simulink model "OMSv1_3"  (Simulink 6.6)
settings: Solver=ode4  SolverMode=SingleTasking  StartTime=0.0  StopTime=9  FixedStep=0.001  MaxStep=0.001  RelTol=1e-3  AbsTol=1e-3
undefined symbols (not defined in the file): alexlaw, bs_onoff, bs_scale, bsfsacrit, bsfsvcrit, cnsgain, fs_onoff, fs_scale, fsdelaycalc, ltdrk, phasicgain, pmcgain, pmctau2, pmctau3, saccsw, spgain, tonicgain, tvrD, tvrN
(part 2 of 7)

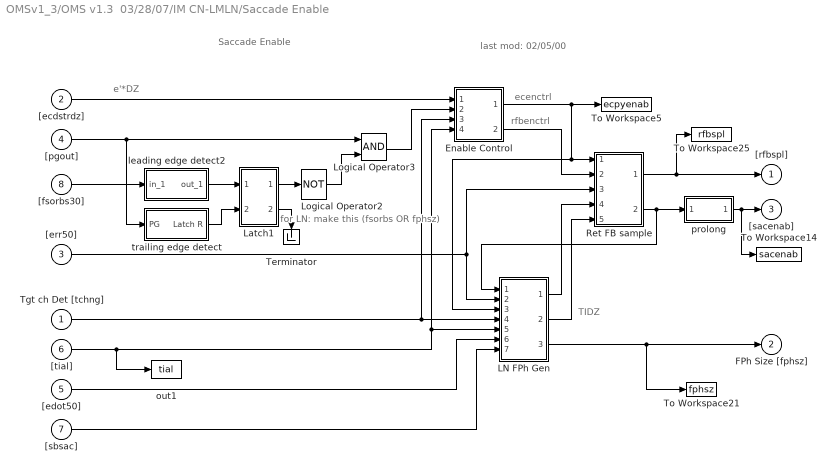
== system OMSv1_3/OMS v1.3  03/28/07/IM CN-LMLN/Saccade Enable ==
  note: Saccade Enable
  note: last mod:
      | 02/05/00
  note: rfbenctrl
  note: ecenctrl
  note: e'*DZ
  note: for LN: make this
      | (fsorbs OR fphsz)
  note: TIDZ
  Tgt ch Det [tchng] : Inport
  "[ecdstrdz]" : Inport  Port=2
  "[err50]" : Inport  Port=3
  "[pgout]" : Inport  Port=4
  "[edot50]" : Inport  Port=5
  "[tial]" : Inport  Port=6
  "[sbsac]" : Inport  Port=7
  "[fsorbs30]" : Inport  Port=8
  Enable Control : Subsystem
      mask Display: disp('Enable\nControl')
  LN FPh Gen : Subsystem
      mask Display: disp('DFFPh\nGen')
  Latch1 : Subsystem  mask(Latch){@1=0}
      mask prompts: @1 "Initial State for Output "Q":"
      mask help: Latch
      mask init:
      | ini=(@1~=0);
      mask Help: Latches the S input.  When S (set) is one, the Q output  becomes one.  The output remains one until the R (reset) input becomes one, forcing the output to zero.  If both R and S are one, the latch will be in an undefined state.
      mask Display: disp('S   Q\n\nR  !Q')
  Logical Operator2 : Logic  Operator=NOT  Inputs=1
  Logical Operator3 : Logic
  Ret FB sample : Subsystem
      mask Display: disp('Ret FB\nEnab &\nSample')
  Terminator : Terminator
      settings: Orientation=down
  To Workspace14 : ToWorkspace  VariableName=sacenab  SaveFormat=Array
      settings: MaxDataPoints=10000
      mask Type: imsw1in
  To Workspace21 : ToWorkspace  VariableName=fphsz  SaveFormat=Array
      settings: MaxDataPoints=10000
  To Workspace25 : ToWorkspace  VariableName=rfbspl  SaveFormat=Array
      settings: MaxDataPoints=10000
      mask Type: imsw1in
  To Workspace5 : ToWorkspace  VariableName=ecpyenab  SaveFormat=Array
      settings: MaxDataPoints=10000
      mask Type: imsw1in
  leading edge detect2 : Subsystem
      mask Display: disp('Leading\nEdge Det')
  out1 : ToWorkspace  VariableName=tial  SaveFormat=Array
      settings: MaxDataPoints=100000
  prolong : Subsystem  mask{prolong=10}
      mask prompts: prolong "Prolong pulse by?  (msec)"
      mask Display: disp('prolong')
  trailing edge detect : Subsystem
      mask Display: disp('Trailing\nEdge Det')
  "[rfbspl]" : Outport  InitialOutput=0
  FPh Size [fphsz] : Outport  Port=2  InitialOutput=0
  "[sacenab]" : Outport  Port=3  InitialOutput=0
  wires:
  "[pgout]"/1 -> Logical Operator3/1, trailing edge detect/1(PG)
  Logical Operator2/1 -> Logical Operator3/2
  "[ecdstrdz]"/1 -> Enable Control/1(e'*DZ [ecdstrdz])
  Tgt ch Det [tchng]/1 -> LN FPh Gen/4(TCD [tchng]), Enable Control/3(Tgt ch Det [tchng])
  "[sbsac]"/1 -> LN FPh Gen/7("[sbsac]")
  "[edot50]"/1 -> LN FPh Gen/6("[edot50]")
  Enable Control/1(ECPY EnTmng [ecpyenab]) -> LN FPh Gen/3("[ecpyenab]"), Ret FB sample/1("[ecpyenab]"), To Workspace5/1
  "[err50]"/1 -> LN FPh Gen/2("[err50]"), Ret FB sample/3("[err50]")
  Enable Control/2(RetFB En&Spl) -> Ret FB sample/2("[rfbenctrl]")
  LN FPh Gen/2(TIDZ) -> Ret FB sample/5(TIDZ)
  Ret FB sample/2(RetFB Enable [sacenab]) -> prolong/1(value(in)), LN FPh Gen/1("[rfbenab]")
  "[fsorbs30]"/1 -> leading edge detect2/1(in_1)
  leading edge detect2/1(out_1) -> Latch1/1(in_1)
  Latch1/1(out_1) -> Logical Operator2/1
  trailing edge detect/1(Latch R) -> Latch1/2(in_2)
  Logical Operator3/1 -> Enable Control/2(VolPG ( [pgout] &NOT fs or bs))
  LN FPh Gen/1("[eedot]") -> Ret FB sample/4("[eedot]")
  Ret FB sample/1(RFB Spl [rfbspl]) -> "[rfbspl]"/1, To Workspace25/1
  LN FPh Gen/3(FPh Size [fphsz]) -> FPh Size [fphsz]/1, To Workspace21/1
  prolong/1(value(out)) -> "[sacenab]"/1, To Workspace14/1
  "[tial]"/1 -> LN FPh Gen/5("[tial]"), Enable Control/4("[tial]"), out1/1
  Latch1/2(out_2) -> Terminator/1

== system OMSv1_3/OMS v1.3  03/28/07/IM CN-LMLN/Saccade Motor Commmand ==
  note: last mod:
      | 02/25/01
  note: Saccadic Motor Command
  note: If TCHNG occurs, BLOCK
      | BS/FS (and already prog vs?)
      | for 150 msec
  note: If TCHNG occurs:
      | ALLOW vol sacc
  note: make sure that tchngOVR
      | lets _something_ pass,
      | since it operates switches
      | in two different locations...
  "[ecdstrdz]" : Inport
  "[fphsz]" : Inport  Port=2
  Tgt ch Det [tchng] : Inport  Port=3
  "[sacenab]" : Inport  Port=4
  "[fsorbs30]" : Inport  Port=5
  "[fsbcmc30]" : Inport  Port=6
  "\"slip vel\"1" : Sum  SaturateOnIntegerOverflow=on  InputSameDT=on
  (0.5) : Switch  Threshold=.5  SaturateOnIntegerOverflow=on  InputSameDT=on
  0 : Constant  Orientation=left  Value=0
  Switch3 : Switch  Threshold=.5  SaturateOnIntegerOverflow=on  InputSameDT=on
  TCHNG Override : Subsystem
      mask Display: disp('TCHNG\nOverride')
  To Workspace30 : ToWorkspace  VariableName=fsbsmc30  SaveFormat=Array
      settings: MaxDataPoints=10000
  To Workspace6 : ToWorkspace  VariableName=posmc  SaveFormat=Array
      settings: MaxDataPoints=10000
  Voluntary Saccade Switch : Subsystem
      mask Display: disp('Vol\nSacc\nSw')
  timer value : Constant  Orientation=left  Value=0.15
  "[posmc]" : Outport  InitialOutput=0
  wires:
  "[ecdstrdz]"/1 -> "\"slip vel\"1"/1
  "[fphsz]"/1 -> "\"slip vel\"1"/2
  "[sacenab]"/1 -> Voluntary Saccade Switch/2("[sacenab]")
  0/1 -> Switch3/3
  (0.5)/1 -> Switch3/1
  "[fsorbs30]"/1 -> Voluntary Saccade Switch/3("[fsorbs30]")
  Voluntary Saccade Switch/2(sacenab/0) -> (0.5)/2
  Tgt ch Det [tchng]/1 -> TCHNG Override/1("[tchng]")
  timer value/1 -> TCHNG Override/2(timer dur)
  "\"slip vel\"1"/1 -> Voluntary Saccade Switch/1("[fphmag]")
  Voluntary Saccade Switch/1("[vsmc]") -> (0.5)/1
  TCHNG Override/1(tchng sw) -> Switch3/2
  "[fsbcmc30]"/1 -> (0.5)/3, To Workspace30/1
  Switch3/1 -> "[posmc]"/1, To Workspace6/1

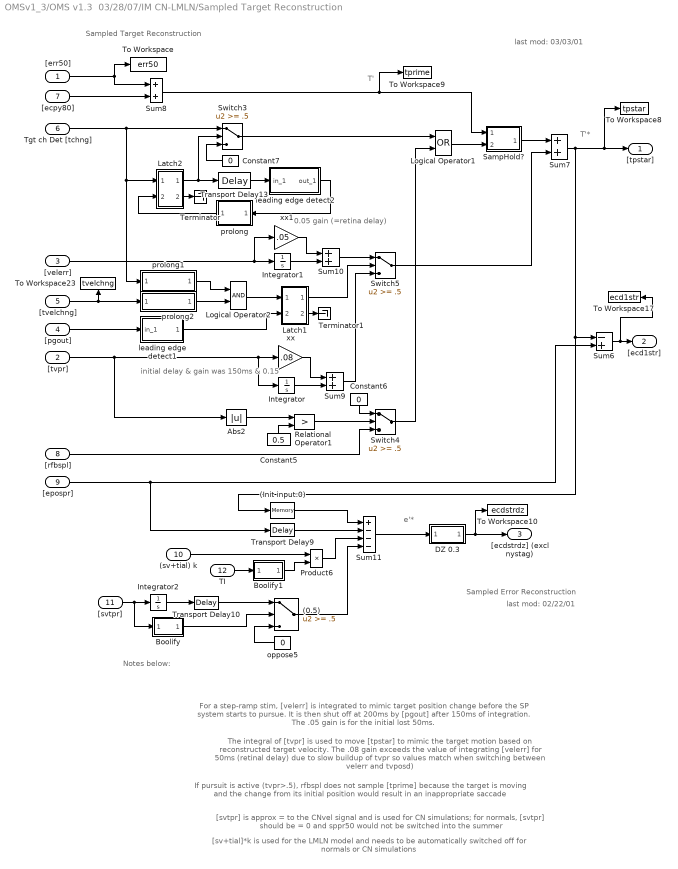
== system OMSv1_3/OMS v1.3  03/28/07/IM CN-LMLN/Sampled Target Reconstruction ==
  note: T'
  note: T'*
  note: Sampled Target Reconstruction
  note: last mod:
      | 03/03/01
  note: Notes below:
  note: If pursuit is active (tvpr>.5), rfbspl does not sample [tprime] because the target is moving and
      | the change from its initial position would result in an inappropriate saccade
  note: The integral of [tvpr] is used to move [tpstar] to mimic the target motion based on reconstructed target velocity. The .08 gain
      | exceeds the value of integrating [velerr] for 50ms (retinal delay) due to slow buildup of tvpr so values match
      | when switching between velerr and tvposd)
  note: For a step-ramp stim, [velerr] is integrated to mimic target position change before the SP system starts to pursue.
      |  It is then shut off at 200ms by [pgout] after 150ms of integration. The .05 gain is for the initial lost 50ms.
  note: initial delay & gain
      | was 150ms & 0.15
  note: 0.05 gain (=retina delay)
  note: e'*
  note: Sampled Error Reconstruction
  note: last mod:
      | 02/22/01
  note: [svtpr] is approx = to the CNvel signal and is used for CN simulations; for normals, [svtpr]
      | should be = 0 and sppr50 would not be switched into the summer
  note: [sv+tial]*k is used for the LMLN model and needs to be automatically switched off
      | for normals or CN simulations
  "[err50]" : Inport
  "[tvpr]" : Inport  Port=2
  "[velerr]" : Inport  Port=3
  "[pgout]" : Inport  Port=4
  "[tvelchng]" : Inport  Port=5
  Tgt ch Det [tchng] : Inport  Port=6
  "[ecpy80]" : Inport  Port=7
  "[rfbspl]" : Inport  Port=8
  "[epospr]" : Inport  Port=9
  (sv+tial) k : Inport  Port=10
  "[svtpr]" : Inport  Port=11
  TI : Inport  Port=12
  (0.5) : Switch  Threshold=.5  SaturateOnIntegerOverflow=on  InputSameDT=on
  (Init input:0) : Memory
  Abs2 : Abs  SaturateOnIntegerOverflow=on
  Boolify : Subsystem
      mask Display: disp('Boolify')
  Boolify1 : Subsystem
      mask Display: disp('Boolify')
  Constant5 : Constant  Orientation=up  Value=0.5
  Constant6 : Constant  Orientation=down  Value=0
  Constant7 : Constant  Orientation=left  Value=0
  DZ 0.3 : Subsystem
      mask Display: disp('DZ 0.3')
  Integrator : Integrator
  Integrator1 : Integrator
  Integrator2 : Integrator
  Latch1 : Subsystem  mask(Latch){@1=0}
      mask prompts: @1 "Initial State for Output "Q":"
      mask help: Latch
      mask init:
      | ini=(@1~=0);
      mask Help: Latches the S input.  When S (set) is one, the Q output  becomes one.  The output remains one until the R (reset) input becomes one, forcing the output to zero.  If both R and S are one, the latch will be in an undefined state.
      mask Display: disp('S   Q\n\nR  !Q')
  Latch2 : Subsystem  mask(Latch){@1=0}
      mask prompts: @1 "Initial State for Output "Q":"
      mask help: Latch
      mask init:
      | ini=(@1~=0);
      mask Help: Latches the S input.  When S (set) is one, the Q output  becomes one.  The output remains one until the R (reset) input becomes one, forcing the output to zero.  If both R and S are one, the latch will be in an undefined state.
      mask Display: disp('S   Q\n\nR  !Q')
  Logical Operator1 : Logic  Operator=OR
  Logical Operator2 : Logic
  Product6 : Product  SaturateOnIntegerOverflow=on  RndMeth=Zero  InputSameDT=on
  Relational Operator1 : RelationalOperator  Operator=>  InputSameDT=on
  SampHold? : Subsystem
      mask Display: disp('S=H\nH=L')
  Sum{7..10} (4 alike) : Sum  SaturateOnIntegerOverflow=on  InputSameDT=on
  Sum11 : Sum  Inputs=+---  SaturateOnIntegerOverflow=on  InputSameDT=on
  Sum6 : Sum  Inputs=-+  SaturateOnIntegerOverflow=on  InputSameDT=on
  Switch3 : Switch  Threshold=.5  SaturateOnIntegerOverflow=on  InputSameDT=on
  Switch4 : Switch  Threshold=.5  SaturateOnIntegerOverflow=on  InputSameDT=on
  Switch5 : Switch  Threshold=.5  SaturateOnIntegerOverflow=on  InputSameDT=on
  Terminator : Terminator
  Terminator1 : Terminator
  To Workspace : ToWorkspace  VariableName=err50  SaveFormat=Array
      settings: MaxDataPoints=10000
  To Workspace10 : ToWorkspace  VariableName=ecdstrdz  SaveFormat=Array
      settings: MaxDataPoints=10000
  To Workspace17 : ToWorkspace  VariableName=ecd1str  SaveFormat=Array
      settings: MaxDataPoints=10000
  To Workspace23 : ToWorkspace  VariableName=tvelchng  SaveFormat=Array
      settings: Orientation=up  MaxDataPoints=10000
  To Workspace8 : ToWorkspace  VariableName=tpstar  SaveFormat=Array
      settings: MaxDataPoints=10000
  To Workspace9 : ToWorkspace  VariableName=tprime  SaveFormat=Array
      settings: MaxDataPoints=10000
  Transport Delay10 : TransportDelay  DelayTime=.05
      mask Display: disp('50ms')
  Transport Delay13 : TransportDelay  DelayTime=.05
      mask Display: disp('50ms')
  Transport Delay9 : TransportDelay  DelayTime=.05
      mask Display: disp('50ms')
  leading edge detect1 : Subsystem
      mask Display: disp('Leading\nEdge Det')
  leading edge detect2 : Subsystem
      mask Display: disp('Leading\nEdge Det')
  oppose5 : Constant  Orientation=left  Value=0
  prolong : Subsystem  Orientation=left  mask{prolong=150}
      mask prompts: prolong "Prolong pulse by?  (msec)"
      mask Display: disp('150ms\nprolong')
  prolong1 : Subsystem  mask{prolong=5}
      mask prompts: prolong "Prolong pulse by?  (msec)"
      mask Display: disp('5ms prolong')
  prolong2 : Subsystem  mask{prolong=5}
      mask prompts: prolong "Prolong pulse by?  (msec)"
      mask Display: disp('5ms prolong')
  xx : Gain  Gain=.08  SaturateOnIntegerOverflow=on
  xx1 : Gain  Gain=.05  SaturateOnIntegerOverflow=on
  "[tpstar]" : Outport  InitialOutput=0
  "[ecd1str]" : Outport  Port=2  InitialOutput=0
  "[ecdstrdz] (excl nystag)" : Outport  Port=3  InitialOutput=0
  wires:
  Sum8/1 -> To Workspace9/1, SampHold?/1(Input)
  "[ecpy80]"/1 -> Sum8/2
  prolong1/1(value(out)) -> Logical Operator2/1
  Tgt ch Det [tchng]/1 -> Switch3/1, Latch2/1(in_1), prolong1/1(value(in))
  Logical Operator1/1 -> SampHold?/2(S/H?)
  Sum7/1 -> Sum6/1, (Init input:0)/1, "[tpstar]"/1, To Workspace8/1
  SampHold?/1(output) -> Sum7/1
  Switch3/1 -> Logical Operator1/1
  Constant7/1 -> Switch3/3
  Latch2/1(out_1) -> Switch3/2, Transport Delay13/1
  Transport Delay13/1 -> leading edge detect2/1(in_1)
  leading edge detect2/1(out_1) -> prolong/1(value(in))
  prolong/1(value(out)) -> Latch2/2(in_2)
  Sum10/1 -> Switch5/1
  Integrator1/1 -> Sum10/2
  xx1/1 -> Sum10/1
  Abs2/1 -> Relational Operator1/1
  Constant6/1 -> Switch4/1
  Constant5/1 -> Relational Operator1/2
  Relational Operator1/1 -> Switch4/2
  "[rfbspl]"/1 -> Switch4/3
  Integrator/1 -> Sum9/2
  xx/1 -> Sum9/1
  "[tvpr]"/1 -> Abs2/1, xx/1, Integrator/1
  Switch4/1 -> Logical Operator1/2
  leading edge detect1/1(out_1) -> Latch1/2(in_2)
  "[pgout]"/1 -> leading edge detect1/1(in_1)
  Logical Operator2/1 -> Latch1/1(in_1)
  prolong2/1(value(out)) -> Logical Operator2/2
  "[velerr]"/1 -> Integrator1/1, xx1/1
  Switch5/1 -> Sum7/2
  Latch1/1(out_1) -> Switch5/2
  Sum9/1 -> Switch5/3
  "[epospr]"/1 -> Sum6/2, Transport Delay9/1
  "[tvelchng]"/1 -> prolong2/1(value(in)), To Workspace23/1
  Sum6/1 -> "[ecd1str]"/1, To Workspace17/1
  "[err50]"/1 -> Sum8/1, To Workspace/1
  TI/1 -> Boolify1/1(In1)
  Boolify1/1(Out1) -> Product6/2
  (sv+tial) k/1 -> Product6/1
  Product6/1 -> Sum11/3
  oppose5/1 -> (0.5)/3
  "[svtpr]"/1 -> Integrator2/1, Boolify/1(In1)
  Boolify/1(Out1) -> (0.5)/2
  (Init input:0)/1 -> Sum11/1
  Transport Delay9/1 -> Sum11/2
  Sum11/1 -> DZ 0.3/1(in_1)
  Transport Delay10/1 -> (0.5)/1
  (0.5)/1 -> Sum11/4
  Integrator2/1 -> Transport Delay10/1
  DZ 0.3/1(out_1) -> "[ecdstrdz] (excl nystag)"/1, To Workspace10/1
  Latch2/2(out_2) -> Terminator/1
  Latch1/2(out_2) -> Terminator1/1

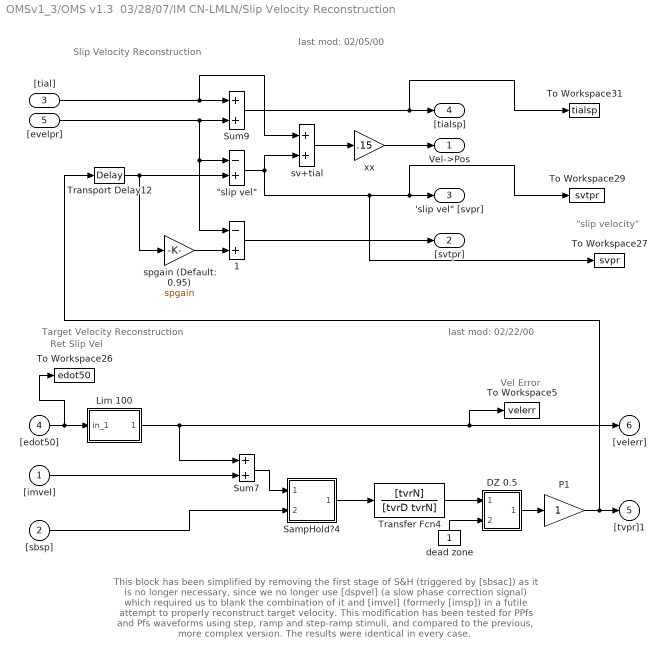
== system OMSv1_3/OMS v1.3  03/28/07/IM CN-LMLN/Slip Velocity Reconstruction ==
  note: last mod:
      | 02/05/00
  note: Slip Velocity Reconstruction
  note: last mod:
      | 02/22/00
  note: Target Velocity Reconstruction
  note: This block has been simplified by removing the first stage of S&H (triggered by [sbsac]) as it is no longer necessary,
      | since we no longer use [dspvel] (a slow phase correction signal) which required us to blank the combination of it
      | and [imvel] (formerly [imsp]) in a futile attempt to properly reconstruct target velocity.  This modification has been tested
      | for PPfs and Pfs waveforms using step, ramp and step-ramp stimuli, and compared to the previous, more complex
      | version.  The results were identical in every case.
  note: "slip velocity"
  note: Vel
      | Error
  note: Ret Slip Vel
  "[imvel]" : Inport
  "[sbsp]" : Inport  Port=2
  "[tial]" : Inport  Port=3
  "[edot50]" : Inport  Port=4
  "[evelpr]" : Inport  Port=5
  " 1" : Sum  Inputs=-+  SaturateOnIntegerOverflow=on  InputSameDT=on
  "\"slip vel\"" : Sum  Inputs=-+  SaturateOnIntegerOverflow=on  InputSameDT=on
  DZ 0.5 : Subsystem
      mask Display: disp('Dead\nZone')
  Lim 100 : Subsystem
      mask Display: disp('Limiter')
  P1 : Gain  SaturateOnIntegerOverflow=on
  SampHold?4 : Subsystem
      mask Display: disp('S=H\nH=L')
  Sum7 : Sum  SaturateOnIntegerOverflow=on  InputSameDT=on
  Sum9 : Sum  SaturateOnIntegerOverflow=on  InputSameDT=on
  To Workspace26 : ToWorkspace  VariableName=edot50  SaveFormat=Array
      settings: MaxDataPoints=10000
  To Workspace27 : ToWorkspace  VariableName=svpr  SaveFormat=Array
      settings: MaxDataPoints=10000
  To Workspace29 : ToWorkspace  VariableName=svtpr  SaveFormat=Array
      settings: MaxDataPoints=10000
  To Workspace31 : ToWorkspace  VariableName=tialsp  SaveFormat=Array
      settings: MaxDataPoints=10000
  To Workspace5 : ToWorkspace  VariableName=velerr  SaveFormat=Array
      settings: MaxDataPoints=10000
  Transfer Fcn4 : TransferFcn  Numerator=[tvrN]  Denominator=[tvrD tvrN]
  Transport Delay12 : TransportDelay  DelayTime=.05
      mask Display: disp('50ms')
  dead zone : Constant  Orientation=up
  spgain (Default: 0.95) : Gain  Gain=spgain  SaturateOnIntegerOverflow=on
  sv+tial : Sum  SaturateOnIntegerOverflow=on  InputSameDT=on
  xx : Gain  Gain=.15  SaturateOnIntegerOverflow=on
  Vel->Pos : Outport  InitialOutput=0
  "[svtpr]" : Outport  Port=2  InitialOutput=0
  "'slip vel\" [svpr]" : Outport  Port=3  InitialOutput=0
  "[tialsp]" : Outport  Port=4  InitialOutput=0
  "[tvpr]1" : Outport  Port=5  InitialOutput=0
  "[velerr]" : Outport  Port=6  InitialOutput=0
  wires:
  xx/1 -> Vel->Pos/1
  sv+tial/1 -> xx/1
  "[tial]"/1 -> sv+tial/1, Sum9/1
  "\"slip vel\""/1 -> sv+tial/2, To Workspace27/1, "'slip vel\" [svpr]"/1, To Workspace29/1
  "[evelpr]"/1 -> Sum9/2, "\"slip vel\""/1, " 1"/1
  spgain (Default: 0.95)/1 -> " 1"/2
  " 1"/1 -> "[svtpr]"/1
  Transport Delay12/1 -> "\"slip vel\""/2, spgain (Default: 0.95)/1
  dead zone/1 -> DZ 0.5/2(in_2)
  DZ 0.5/1(out_1) -> P1/1
  "[sbsp]"/1 -> SampHold?4/2(S/H?)
  "[imvel]"/1 -> Sum7/2
  Lim 100/1(out_1) -> Sum7/1, "[velerr]"/1, To Workspace5/1
  Sum7/1 -> SampHold?4/1(Input)
  SampHold?4/1(output) -> Transfer Fcn4/1
  Transfer Fcn4/1 -> DZ 0.5/1(in_1)
  Sum9/1 -> "[tialsp]"/1, To Workspace31/1
  "[edot50]"/1 -> Lim 100/1(in_1), To Workspace26/1
  P1/1 -> "[tvpr]1"/1, Transport Delay12/1

== system OMSv1_3/OMS v1.3  03/28/07/IM CN-LMLN/Target Change Detection ==
  note: Target Change Detection
  note: Detects T change >1 deg any time
  RetErr Vel [edot50] : Inport
  "[tvpr]" : Inport  Port=2
  Abs2 : Abs  SaturateOnIntegerOverflow=on
  Abs3 : Abs  SaturateOnIntegerOverflow=on
  Constant5 : Constant  Orientation=up  Value=950
  Constant6 : Constant  Orientation=up  Value=950
  Derivative : Derivative
      mask Display: disp('s')
  Relational Operator : RelationalOperator  InputSameDT=on
  Relational Operator1 : RelationalOperator  InputSameDT=on
  To Workspace20 : ToWorkspace  VariableName=tchng  SaveFormat=Array
      settings: MaxDataPoints=10000
  Tvel Chng [tvelchng] : Outport  InitialOutput=0
  Trgt Chng [tchng] : Outport  Port=2  InitialOutput=0
  wires:
  RetErr Vel [edot50]/1 -> Abs2/1
  Constant5/1 -> Relational Operator/2
  Abs2/1 -> Relational Operator/1
  Constant6/1 -> Relational Operator1/2
  Abs3/1 -> Relational Operator1/1
  "[tvpr]"/1 -> Derivative/1
  Derivative/1 -> Abs3/1
  Relational Operator1/1 -> Tvel Chng [tvelchng]/1
  Relational Operator/1 -> Trgt Chng [tchng]/1, To Workspace20/1

== system OMSv1_3/OMS v1.3  03/28/07/IM CN-LMLN/setmdlp ==

== system OMSv1_3/OMS v1.3  03/28/07/OMN2/SampHold? ==
  note: When "S/H?" is LOW, then "Input" is switched directly to the
      | output ("sample").  When "S/H?" is HIGH, the current output is
      | maintained ("hold").
  Input : Inport
  S/H? : Inport  Port=2
  Memory : Memory  Orientation=left
  Sign : Subsystem
      mask Type: Sign
      mask Description: y = sign(x)
      mask Help: Sign Function:\n\t\t\ty = 1 if x > 0\n\t\t\ty = 0 if x = 0\n\t\t\ty = -1 if x < 0
      mask Display: plot(-50,-50,50,50,[-50,50],[0,0],[0,0],[-50,50],[-40,0],[-30,-30],[0,40],[30,30])
  Switch2 : Switch  Threshold=0.5  SaturateOnIntegerOverflow=on  InputSameDT=on
  output : Outport  InitialOutput=0
  wires:
  Switch2/1 -> Memory/1, output/1
  Memory/1 -> Switch2/1
  Input/1 -> Switch2/3
  Sign/1(out_1) -> Switch2/2
  S/H?/1 -> Sign/1(in_1)

== system OMSv1_3/OMS v1.3  03/28/07/OMN2/Sign ==
  in_1 : Inport
  Constant : Constant  Value=0
  Relational Operator : RelationalOperator  Operator=>  InputSameDT=on
  Relational Operator1 : RelationalOperator  Operator=<  InputSameDT=on
  Sum : Sum  Inputs=+-  SaturateOnIntegerOverflow=on  InputSameDT=on
  out_1 : Outport  InitialOutput=0
  wires:
  Sum/1 -> out_1/1
  Relational Operator/1 -> Sum/1
  Relational Operator1/1 -> Sum/2
  Constant/1 -> Relational Operator1/2, Relational Operator/2
  in_1/1 -> Relational Operator/1, Relational Operator1/1

== system OMSv1_3/OMS v1.3  03/28/07/OMS model lib/plantlib link ==

== system OMSv1_3/OMS v1.3  03/28/07/OMS model lib/plantlib link1 ==

== system OMSv1_3/OMS v1.3  03/28/07/OMS model lib/plantlib link2 ==

== system OMSv1_3/OMS v1.3  03/28/07/OMS model lib/plantlib link3 ==

== system OMSv1_3/OMS v1.3  03/28/07/OMS model lib/plantlib link4 ==

== system OMSv1_3/OMS v1.3  03/28/07/OMS model lib/plantlib link5 ==

== system OMSv1_3/OMS v1.3  03/28/07/OMS model lib/plantlib link6 ==

== system OMSv1_3/OMS v1.3  03/28/07/OMS model lib/plantlib link7 ==

== system OMSv1_3/OMS v1.3  03/28/07/OMS model lib/stimlib ==

== system OMSv1_3/OMS v1.3  03/28/07/PG w rNI1/PW funct ==
  note: This process continues until the error has been driven to zero or the input drops to zero,
      | and the integrator is reset and the pulse is ended.
  note: The input, scaled by the piece-wise linear function, is compared to the output of the
      | resettable integrator, which integrates a constant value each iteration.
  note: This block uses a resettable integrator and a piecewise-linear function (PWfunc) to generate
      | a pulse of appropriate duration for the incoming stimulus.
  note: (Init input:0)
  note: PW Function
  mcspl : Inport
  Abs : Abs  SaturateOnIntegerOverflow=on
  Constant1 : Constant  Orientation=up  Value=0
  Constant3 : Constant  Orientation=down  Value=1000
  Good Reset Integrator2 : Subsystem  Orientation=left
      mask Display: disp('Resettable\nNI')
  Input Switch : Subsystem
      mask Display: disp('Input\nSwitch')
  Logical Operator : Logic  Orientation=left  Operator=OR
  Logical Operator1 : Logic  Orientation=up  Operator=NOT  Inputs=1
  PWfn : Lookup  Orientation=down  InputValues=[ 0, 0.1:5, 5:10, 10:50 ]  OutputValues="[ 0, (0.1:5)*0+15,  (5:10)*1+10,  (10:50)*2]"  SaturateOnIntegerOverflow=on
  Relational Operator1 : RelationalOperator  InputSameDT=on
  Relational Operator2 : RelationalOperator  Operator=<=  InputSameDT=on
  Sign : Subsystem
      mask Type: Sign
      mask Description: y = sign(x)
      mask Help: Sign Function:\n\t\t\ty = 1 if x > 0\n\t\t\ty = 0 if x = 0\n\t\t\ty = -1 if x < 0
      mask Display: plot(-50,-50,50,50,[-50,50],[0,0],[0,0],[-50,50],[-40,0],[-30,-30],[0,40],[30,30])
  Sum : Sum  Inputs=-+  SaturateOnIntegerOverflow=on  InputSameDT=on
  dead zone : Constant  Orientation=up  Value=.04
  loop breaker : Memory  Orientation=left
  out thresh : Constant  Value=0.2
  pgw : Outport  InitialOutput=0
  wires:
  Logical Operator1/1 -> Logical Operator/2
  Relational Operator1/1 -> Logical Operator1/1, Sign/1(in_1)
  Constant3/1 -> Good Reset Integrator2/1(input)
  Constant1/1 -> Good Reset Integrator2/3(initial condition)
  out thresh/1 -> Relational Operator1/2
  Input Switch/1(mcsw) -> Abs/1
  mcspl/1 -> Input Switch/1(mcspl)
  Sign/1(out_1) -> pgw/1, loop breaker/1
  Abs/1 -> PWfn/1, Relational Operator2/1
  PWfn/1 -> Sum/2
  Sum/1 -> Relational Operator1/1
  Logical Operator/1 -> Good Reset Integrator2/2(reset?)
  Good Reset Integrator2/1(out_1) -> Sum/1
  dead zone/1 -> Relational Operator2/2
  Relational Operator2/1 -> Logical Operator/1
  loop breaker/1 -> Input Switch/2(pgw)

== system OMSv1_3/OMS v1.3  03/28/07/PG w rNI1/RefLatch (Default = 50ms) ==
  note: It's a cheap trick, but it seems to work:
  note: The falling edge" block's output becomes DISABLED upon
      | detection of the END of the input pulse, and remains
      | so until the refractory period of rp milliseconds has elapsed.
  note: By ANDing these outputs, we get a signal that is DISABLED
      | starting with the beginning of the input pulse, and remains so until
      | rp milliseconds after the termination of the pulse.
  note: The "NOT" gate outputs a DISABLE signal whenever there is any
      | input, so that there can be no response.
  in_1 : Inport
  Abs : Abs  SaturateOnIntegerOverflow=on
  Logical Operator : Logic
  Logical Operator1 : Logic  Operator=NOT  Inputs=1
  trailing edge : Subsystem
      mask Display: disp('Refract\nLatch (te)')
  out_1 : Outport  InitialOutput=0
  wires:
  Logical Operator/1 -> out_1/1
  Logical Operator1/1 -> Logical Operator/1
  trailing edge/1(out_1) -> Logical Operator/2
  Abs/1 -> Logical Operator1/1, trailing edge/1(in_1)
  in_1/1 -> Abs/1

== system OMSv1_3/OMS v1.3  03/28/07/PG w rNI1/SampHold?1 ==
  note: When "S/H?" is HIGH, then "Input" is switched directly to the
      | output ("sample").  When "S/H?" is LOW, the current output is
      | maintained ("hold").
  Input : Inport
  S/H? : Inport  Port=2
  Memory : Memory  Orientation=left
  Sign : Subsystem
      mask Type: Sign
      mask Description: y = sign(x)
      mask Help: Sign Function:\n\t\t\ty = 1 if x > 0\n\t\t\ty = 0 if x = 0\n\t\t\ty = -1 if x < 0
      mask Display: plot(-50,-50,50,50,[-50,50],[0,0],[0,0],[-50,50],[-40,0],[-30,-30],[0,40],[30,30])
  Switch2 : Switch  Threshold=0.5  SaturateOnIntegerOverflow=on  InputSameDT=on
  output : Outport  InitialOutput=0
  wires:
  S/H?/1 -> Sign/1(in_1)
  Sign/1(out_1) -> Switch2/2
  Input/1 -> Switch2/1
  Switch2/1 -> output/1, Memory/1
  Memory/1 -> Switch2/3

== system OMSv1_3/OMS v1.3  03/28/07/Fixation/30 /Latch1 ==
  in_1 : Inport
  in_2 : Inport  Port=2
  Demux : Demux  Outputs=2
  Logic : CombinatorialLogic  TruthTable=[0 1;0 1;1 0;0 1;1 0;0 1;1 0;1 0]
  Memory : Memory  Orientation=left  X0=ini
  Mux : Mux  Inputs=3
  out_1 : Outport  InitialOutput=0
  out_2 : Outport  Port=2  InitialOutput=0
  wires:
  in_2/1 -> Mux/3
  in_1/1 -> Mux/2
  Memory/1 -> Mux/1
  Demux/1 -> Memory/1, out_1/1
  Mux/1 -> Logic/1
  Logic/1 -> Demux/1
  Demux/2 -> out_2/1

== system OMSv1_3/OMS v1.3  03/28/07/Fixation/30 /SampHold?2 ==
  note: When "S/H?" is LOW, then "Input" is switched directly to the
      | output ("sample").  When "S/H?" is HIGH, the current output is
      | maintained ("hold").
  Input : Inport
  S/H? : Inport  Port=2
  Memory : Memory  Orientation=left
  Sign : Subsystem
      mask Type: Sign
      mask Description: y = sign(x)
      mask Help: Sign Function:\n\t\t\ty = 1 if x > 0\n\t\t\ty = 0 if x = 0\n\t\t\ty = -1 if x < 0
      mask Display: plot(-50,-50,50,50,[-50,50],[0,0],[0,0],[-50,50],[-40,0],[-30,-30],[0,40],[30,30])
  Switch2 : Switch  Threshold=0.5  SaturateOnIntegerOverflow=on  InputSameDT=on
  output : Outport  InitialOutput=0
  wires:
  S/H?/1 -> Sign/1(in_1)
  Sign/1(out_1) -> Switch2/2
  Input/1 -> Switch2/3
  Switch2/1 -> Memory/1, output/1
  Memory/1 -> Switch2/1

== system OMSv1_3/OMS v1.3  03/28/07/Fixation/30 /leading edge detect ==
  note: leading edge detection
  in_1 : Inport
  Abs : Abs  SaturateOnIntegerOverflow=on
  Derivative : Derivative
  Relational Operator : RelationalOperator  Operator===  InputSameDT=on
  Sign : Subsystem
      mask Type: Sign
      mask Description: y = sign(x)
      mask Help: Sign Function:\n\t\t\ty = 1 if x > 0\n\t\t\ty = 0 if x = 0\n\t\t\ty = -1 if x < 0
      mask Display: plot(-50,-50,50,50,[-50,50],[0,0],[0,0],[-50,50],[-40,0],[-30,-30],[0,40],[30,30])
  Threshold 1 : Constant
  out_1 : Outport  InitialOutput=0
  wires:
  in_1/1 -> Abs/1
  Relational Operator/1 -> out_1/1
  Threshold 1/1 -> Relational Operator/2
  Sign/1(out_1) -> Relational Operator/1
  Derivative/1 -> Sign/1(in_1)
  Abs/1 -> Derivative/1

== system OMSv1_3/OMS v1.3  03/28/07/Fixation/30 /trailing edge detect ==
  note: It is also possible to remove the SIGNUM function
      | and the '==', and replace them with a simple
      | switch with a threshold of (say) 150 or so.
  note: trailing edge detection
  in_1 : Inport
  Abs : Abs  SaturateOnIntegerOverflow=on
  Derivative : Derivative
  Relational Operator : RelationalOperator  Operator===  InputSameDT=on
  Sign : Subsystem
      mask Type: Sign
      mask Description: y = sign(x)
      mask Help: Sign Function:\n\t\t\ty = 1 if x > 0\n\t\t\ty = 0 if x = 0\n\t\t\ty = -1 if x < 0
      mask Display: plot(-50,-50,50,50,[-50,50],[0,0],[0,0],[-50,50],[-40,0],[-30,-30],[0,40],[30,30])
  Threshold 1 : Constant  Value=-1
  out_1 : Outport  InitialOutput=0
  wires:
  Abs/1 -> Derivative/1
  Derivative/1 -> Sign/1(in_1)
  Sign/1(out_1) -> Relational Operator/1
  Threshold 1/1 -> Relational Operator/2
  Relational Operator/1 -> out_1/1
  in_1/1 -> Abs/1

== system OMSv1_3/OMS v1.3  03/28/07/Fixation/Boolify2/direction1 ==
  in_1 : Inport
  Constant : Constant  Value=0
  Relational Operator : RelationalOperator  Operator=>  InputSameDT=on
  Relational Operator1 : RelationalOperator  Operator=<  InputSameDT=on
  Sum : Sum  Inputs=+-  SaturateOnIntegerOverflow=on  InputSameDT=on
  out_1 : Outport  InitialOutput=0
  wires:
  in_1/1 -> Relational Operator/1, Relational Operator1/1
  Constant/1 -> Relational Operator1/2, Relational Operator/2
  Relational Operator1/1 -> Sum/2
  Relational Operator/1 -> Sum/1
  Sum/1 -> out_1/1

== system OMSv1_3/OMS v1.3  03/28/07/IM CN-LMLN/Alexander's Law/Boolify ==
  TI : Inport
  Abs2 : Abs  SaturateOnIntegerOverflow=on
  direction1 : Subsystem
      mask Type: Sign
      mask Description: y = sign(x)
      mask Help: Sign Function:\n\t\t\ty = 1 if x > 0\n\t\t\ty = 0 if x = 0\n\t\t\ty = -1 if x < 0
      mask Display: plot(-50,-50,50,50,[-50,50],[0,0],[0,0],[-50,50],[-40,0],[-30,-30],[0,40],[30,30])
  Switch Control : Outport  InitialOutput=0
  wires:
  direction1/1(out_1) -> Switch Control/1
  TI/1 -> Abs2/1
  Abs2/1 -> direction1/1(in_1)

== system OMSv1_3/OMS v1.3  03/28/07/IM CN-LMLN/Alexander's Law/Boolify1 ==
  TI : Inport
  Abs2 : Abs  SaturateOnIntegerOverflow=on
  direction1 : Subsystem
      mask Type: Sign
      mask Description: y = sign(x)
      mask Help: Sign Function:\n\t\t\ty = 1 if x > 0\n\t\t\ty = 0 if x = 0\n\t\t\ty = -1 if x < 0
      mask Display: plot(-50,-50,50,50,[-50,50],[0,0],[0,0],[-50,50],[-40,0],[-30,-30],[0,40],[30,30])
  Switch Control : Outport  InitialOutput=0
  wires:
  Abs2/1 -> direction1/1(in_1)
  TI/1 -> Abs2/1
  direction1/1(out_1) -> Switch Control/1

== system OMSv1_3/OMS v1.3  03/28/07/IM CN-LMLN/Alexander's Law/direction ==
  in_1 : Inport
  Constant : Constant  Value=0
  Relational Operator : RelationalOperator  Operator=>  InputSameDT=on
  Relational Operator1 : RelationalOperator  Operator=<  InputSameDT=on
  Sum : Sum  Inputs=+-  SaturateOnIntegerOverflow=on  InputSameDT=on
  out_1 : Outport  InitialOutput=0
  wires:
  in_1/1 -> Relational Operator/1, Relational Operator1/1
  Constant/1 -> Relational Operator1/2, Relational Operator/2
  Relational Operator1/1 -> Sum/2
  Relational Operator/1 -> Sum/1
  Sum/1 -> out_1/1

== system OMSv1_3/OMS v1.3  03/28/07/IM CN-LMLN/BS/FS Logic/BS Enable1 ==
  note: BS Enable
  note: This block allows a BS for up to xx ms (set by "timer value")
      | after the acceleration criterion is met (i.e., drops below threshold)
  note: last mod:
      | 12/08/99
  note: (Default = 40deg/sec^2)
  bsprod : Inport
  "[evelpr]" : Inport  Port=2
  Abs1 : Abs  SaturateOnIntegerOverflow=on
  BS Timing : Subsystem
      mask Display: disp('BS\nEnable\nTiming')
  Derivative : Derivative
      mask Display: disp('s')
  Relational Operator3 : RelationalOperator  Operator=<=  InputSameDT=on
  Switch4 : Switch  Threshold=.5  SaturateOnIntegerOverflow=on  InputSameDT=on
  To Workspace14 : ToWorkspace  VariableName=bscmpr  SaveFormat=Array
      settings: MaxDataPoints=10000
      mask Type: imsw1in
  To Workspace15 : ToWorkspace  VariableName=bsenab  SaveFormat=Array
      settings: MaxDataPoints=10000
      mask Type: imsw1in
  To Workspace16 : ToWorkspace  VariableName=bsaccel1  SaveFormat=Array
      settings: MaxDataPoints=10000
      mask Type: imsw1in
  "accel. thresh " : Constant  Orientation=up  Value=bsfsacrit
  off : Constant  Orientation=up  Value=0
  timer value : Constant  Orientation=up  Value=0.01
  "[bsmc]" : Outport  InitialOutput=0
  wires:
  Relational Operator3/1 -> To Workspace14/1, BS Timing/1(From  <= [cmpr])
  Derivative/1 -> To Workspace16/1, Abs1/1
  Abs1/1 -> Relational Operator3/1
  BS Timing/1("[bsenab]") -> To Workspace15/1, Switch4/2
  "[evelpr]"/1 -> Derivative/1
  off/1 -> Switch4/3
  bsprod/1 -> Switch4/1
  Switch4/1 -> "[bsmc]"/1
  timer value/1 -> BS Timing/2(timer dur)
  "accel. thresh "/1 -> Relational Operator3/2

== system OMSv1_3/OMS v1.3  03/28/07/IM CN-LMLN/BS/FS Logic/FS Enable ==
  note: This block allows a FS for up to xx ms (set by "timer value")
      | after the acceleration criterion is met (i.e., drops below threshold)
  note: FS Enable
  note: last mod:
      | 12/08/99
  note: (Default = 40deg/sec^2)
  fsprod : Inport
  "[evelpr]" : Inport  Port=2
  Abs1 : Abs  SaturateOnIntegerOverflow=on
  Derivative : Derivative
      mask Display: disp('s')
  FS Timing : Subsystem
      mask Display: disp('FS\nEnable\nTiming')
  Relational Operator3 : RelationalOperator  Operator=<=  InputSameDT=on
  SampHold?1 : Subsystem
      mask Display: disp('S=L\nH=H')
  Switch4 : Switch  Threshold=.5  SaturateOnIntegerOverflow=on  InputSameDT=on
  To Workspace16 : ToWorkspace  VariableName=fsaccel  SaveFormat=Array
      settings: MaxDataPoints=10000
      mask Type: imsw1in
  To Workspace17 : ToWorkspace  VariableName=fsenab  SaveFormat=Array
      settings: MaxDataPoints=10000
      mask Type: imsw1in
  accel. thresh : Constant  Orientation=up  Value=bsfsacrit
  off : Constant  Orientation=up  Value=0
  timer value : Constant  Orientation=up  Value=0.01
  "[fsmc]" : Outport  InitialOutput=0
  wires:
  timer value/1 -> FS Timing/2(timer dur)
  accel. thresh/1 -> Relational Operator3/2
  "[evelpr]"/1 -> Derivative/1
  FS Timing/1("[fsenab]") -> Switch4/2, SampHold?1/2(S/H?), To Workspace17/1
  Abs1/1 -> Relational Operator3/1
  Derivative/1 -> Abs1/1, To Workspace16/1
  fsprod/1 -> SampHold?1/1(Input)
  Switch4/1 -> "[fsmc]"/1
  off/1 -> Switch4/3
  SampHold?1/1(output) -> Switch4/1
  Relational Operator3/1 -> FS Timing/1(From  <= [cmpr])

== system OMSv1_3/OMS v1.3  03/28/07/IM CN-LMLN/BS/FS Logic/FS or BS? ==
  note: The position error is compared to its value 3 milliseconds earlier.
      | If the error is _increasing_, we want to make a braking
      | saccade to oppose the runaway.
  note: If the position error is _decreasing_, then the eye is approaching the
      | target, and we would like to generate a foveating saccade, since
      | this is our best time to consider capturing the target.
  note: FS or BS?
  note: use diff & filter?
  pos error [ecd1str] : Inport
  pgout : Inport  Port=2
  Abs : Abs  SaturateOnIntegerOverflow=on
  Boolify : Subsystem
      mask Display: disp('Boolify')
  Relational Operator : RelationalOperator  Operator=>  InputSameDT=on
  SampHold?1 : Subsystem
      mask Display: disp('S&H\n(S=L)\n(H=H)')
  Transport Delay1 : TransportDelay  DelayTime=.002
      mask Display: disp('2ms')
  BS=1 FS=0 : Outport  InitialOutput=0
  wires:
  Transport Delay1/1 -> Relational Operator/2
  pos error [ecd1str]/1 -> Abs/1
  Abs/1 -> Relational Operator/1, Transport Delay1/1
  pgout/1 -> Boolify/1(In1)
  Relational Operator/1 -> SampHold?1/1(Input)
  SampHold?1/1(output) -> BS=1 FS=0/1
  Boolify/1(Out1) -> SampHold?1/2(S/H?)

== system OMSv1_3/OMS v1.3  03/28/07/IM CN-LMLN/BS/FS Logic/TCHNG Override ==
  note: (FF init state: Q=1)
  note: * Leading Edge of input ENABLEs output
  note: Operation:
  note: *FS Enabling is initially DISABLED
  note: * Output of TIMER circuit DISABLES output
  note: TCHNG Override
  "[tchng]" : Inport
  timer dur : Inport  Orientation=up  Port=2
  Latch1 : Subsystem  mask(Latch){@1=1}
      mask prompts: @1 "Initial State for Output "Q":"
      mask help: Latch
      mask init:
      | ini=(@1~=0);
      mask Help: Latches the S input.  When S (set) is one, the Q output  becomes one.  The output remains one until the R (reset) input becomes one, forcing the output to zero.  If both R and S are one, the latch will be in an undefined state.
      mask Display: disp('S   Q\n\nR  !Q')
  Terminator : Terminator
  To Workspace13 : ToWorkspace  VariableName=tchngovr  SaveFormat=Array
      settings: Orientation=down  MaxDataPoints=10000
  event timer2 : Subsystem
      mask Display: disp('Event\nTimer2')
  leading edge detect : Subsystem
      mask Display: disp('Leading\nEdge Det')
  tchng sw : Outport  InitialOutput=0
  wires:
  "[tchng]"/1 -> leading edge detect/1(in_1), event timer2/1(_PG)
  timer dur/1 -> event timer2/2(_timer value (port))
  event timer2/1(out_1) -> Latch1/1(in_1)
  leading edge detect/1(out_1) -> Latch1/2(in_2)
  Latch1/1(out_1) -> tchng sw/1, To Workspace13/1
  Latch1/2(out_2) -> Terminator/1

== system OMSv1_3/OMS v1.3  03/28/07/IM CN-LMLN/BS/FS Logic/direction ==
  in_1 : Inport
  Constant : Constant  Value=0
  Relational Operator : RelationalOperator  Operator=>  InputSameDT=on
  Relational Operator1 : RelationalOperator  Operator=<  InputSameDT=on
  Sum : Sum  Inputs=+-  SaturateOnIntegerOverflow=on  InputSameDT=on
  out_1 : Outport  InitialOutput=0
  wires:
  in_1/1 -> Relational Operator/1, Relational Operator1/1
  Constant/1 -> Relational Operator1/2, Relational Operator/2
  Relational Operator1/1 -> Sum/2
  Relational Operator/1 -> Sum/1
  Sum/1 -> out_1/1

== system OMSv1_3/OMS v1.3  03/28/07/IM CN-LMLN/BS/FS Logic/direction1 ==
  in_1 : Inport
  Constant : Constant  Value=0
  Relational Operator : RelationalOperator  Operator=>  InputSameDT=on
  Relational Operator1 : RelationalOperator  Operator=<  InputSameDT=on
  Sum : Sum  Inputs=+-  SaturateOnIntegerOverflow=on  InputSameDT=on
  out_1 : Outport  InitialOutput=0
  wires:
  in_1/1 -> Relational Operator/1, Relational Operator1/1
  Constant/1 -> Relational Operator1/2, Relational Operator/2
  Relational Operator1/1 -> Sum/2
  Relational Operator/1 -> Sum/1
  Sum/1 -> out_1/1

== system OMSv1_3/OMS v1.3  03/28/07/IM CN-LMLN/BS/FS Logic/prolong ==
  note: init = 0
  note: init = 0
  note: 11/22/99
  note: The start of the input pulse causes the value on input 1 to be held starting when the leading
      | edge occurs, and this value remains latched until 'delay' seconds after the pulse ends (trailing edge).
  note: The one integration step delay before the S&H block's S/H (bottom) input insures
      | that the input value to be latched is available to theS&H block's top input
      | before the S&H block tries to 'hold'.
  note: Stretch the duration of an input pulse, latching it at its value at pulse onset.
  note: init Q = 0
  value(in) : Inport
  " x/1000" : Constant  Orientation=up  Value=0.001
  Latch1 : Subsystem  mask(Latch){@1=0}
      mask prompts: @1 "Initial State for Output "Q":"
      mask help: Latch
      mask init:
      | ini=(@1~=0);
      mask Help: Latches the S input.  When S (set) is one, the Q output  becomes one.  The output remains one until the R (reset) input becomes one, forcing the output to zero.  If both R and S are one, the latch will be in an undefined state.
      mask Display: disp('S   Q\n\nR  !Q')
  Product : Product  SaturateOnIntegerOverflow=on  RndMeth=Zero  InputSameDT=on
  SampHold?2 : Subsystem
      mask Display: disp('S=L\nH=H')
  Terminator : Terminator
      settings: Orientation=down
  Variable Transport Delay : VariableTransportDelay  MaximumDelay=10  MaximumPoints=prolong_buffersize
  leading edge detect : Subsystem
      mask Display: disp('Leading\nEdge Det')
  loop breaker2 : Memory
  stretch : Constant  Value=prolong
  trailing edge detect : Subsystem
      mask Display: disp('Trailing\nEdge Det')
  value(out) : Outport  InitialOutput=0
  wires:
  " x/1000"/1 -> Product/2
  Product/1 -> Variable Transport Delay/2
  stretch/1 -> Product/1
  loop breaker2/1 -> SampHold?2/2(S/H?)
  SampHold?2/1(output) -> value(out)/1
  Latch1/1(out_1) -> loop breaker2/1
  leading edge detect/1(out_1) -> Latch1/1(in_1)
  trailing edge detect/1(out_1) -> Variable Transport Delay/1
  Variable Transport Delay/1 -> Latch1/2(in_2)
  value(in)/1 -> SampHold?2/1(Input), trailing edge detect/1(in_1), leading edge detect/1(in_1)
  Latch1/2(out_2) -> Terminator/1

== system OMSv1_3/OMS v1.3  03/28/07/IM CN-LMLN/MdlPlnt+/OMN2 ==
  note: OMN
  note: Note that the OMN properly combines the pulse with the output of the NI, by latching
      | that output to its value at the moment the pulse appears.
  note: Operation: when [pgout] is active it activates the switch, passing the
      | upper input through to the output.  When the pulse is over, the switch changes,
      | allowing the lower input (from the NI) to pass.
  note: This block behaves like the ocular motor neurons,combining a phasic pulse (from PG)
      | with the tonic step produced by integration of the step, yielding a Pulse-Step
      | to drive the plant.
  "[epossp]" : Inport
  "[pgout]" : Inport  Port=2
  Abs : Abs  SaturateOnIntegerOverflow=on
  Gain _ : Gain  Gain=1.0  SaturateOnIntegerOverflow=on
  SampHold? : Subsystem
      mask Display: disp('S=L\nH=H')
  Sign : Subsystem
      mask Type: Sign
      mask Description: y = sign(x)
      mask Help: Sign Function:\n\t\t\ty = 1 if x > 0\n\t\t\ty = 0 if x = 0\n\t\t\ty = -1 if x < 0
      mask Display: plot(-50,-50,50,50,[-50,50],[0,0],[0,0],[-50,50],[-40,0],[-30,-30],[0,40],[30,30])
  Sum : Sum  SaturateOnIntegerOverflow=on  InputSameDT=on
  Switch : Switch  Threshold=.5  SaturateOnIntegerOverflow=on  InputSameDT=on
  out_1 : Outport  InitialOutput=0
  wires:
  "[epossp]"/1 -> Switch/3, SampHold?/1(Input)
  Sign/1(out_1) -> Switch/2, SampHold?/2(S/H?)
  Gain _/1 -> Sum/1
  SampHold?/1(output) -> Sum/2
  Sum/1 -> Switch/1
  "[pgout]"/1 -> Abs/1, Gain _/1
  Switch/1 -> out_1/1
  Abs/1 -> Sign/1(in_1)

== system OMSv1_3/OMS v1.3  03/28/07/IM CN-LMLN/NI Control/Boolify ==
  In1 : Inport
  Abs2 : Abs  SaturateOnIntegerOverflow=on
  direction1 : Subsystem
      mask Type: Sign
      mask Description: y = sign(x)
      mask Help: Sign Function:\n\t\t\ty = 1 if x > 0\n\t\t\ty = 0 if x = 0\n\t\t\ty = -1 if x < 0
      mask Display: plot(-50,-50,50,50,[-50,50],[0,0],[0,0],[-50,50],[-40,0],[-30,-30],[0,40],[30,30])
  Out1 : Outport  InitialOutput=0
  wires:
  Abs2/1 -> direction1/1(in_1)
  In1/1 -> Abs2/1
  direction1/1(out_1) -> Out1/1

== system OMSv1_3/OMS v1.3  03/28/07/IM CN-LMLN/NI Control/Boolify1 ==
  In1 : Inport
  Abs2 : Abs  SaturateOnIntegerOverflow=on
  direction1 : Subsystem
      mask Type: Sign
      mask Description: y = sign(x)
      mask Help: Sign Function:\n\t\t\ty = 1 if x > 0\n\t\t\ty = 0 if x = 0\n\t\t\ty = -1 if x < 0
      mask Display: plot(-50,-50,50,50,[-50,50],[0,0],[0,0],[-50,50],[-40,0],[-30,-30],[0,40],[30,30])
  Out1 : Outport  InitialOutput=0
  wires:
  direction1/1(out_1) -> Out1/1
  In1/1 -> Abs2/1
  Abs2/1 -> direction1/1(in_1)

== system OMSv1_3/OMS v1.3  03/28/07/IM CN-LMLN/NI Control/Boolify2 ==
  In1 : Inport
  Abs2 : Abs  SaturateOnIntegerOverflow=on
  direction1 : Subsystem
      mask Type: Sign
      mask Description: y = sign(x)
      mask Help: Sign Function:\n\t\t\ty = 1 if x > 0\n\t\t\ty = 0 if x = 0\n\t\t\ty = -1 if x < 0
      mask Display: plot(-50,-50,50,50,[-50,50],[0,0],[0,0],[-50,50],[-40,0],[-30,-30],[0,40],[30,30])
  Out1 : Outport  InitialOutput=0
  wires:
  Abs2/1 -> direction1/1(in_1)
  In1/1 -> Abs2/1
  direction1/1(out_1) -> Out1/1

== system OMSv1_3/OMS v1.3  03/28/07/IM CN-LMLN/NI Control/Boolify3 ==
  In1 : Inport
  Abs2 : Abs  SaturateOnIntegerOverflow=on
  direction1 : Subsystem
      mask Type: Sign
      mask Description: y = sign(x)
      mask Help: Sign Function:\n\t\t\ty = 1 if x > 0\n\t\t\ty = 0 if x = 0\n\t\t\ty = -1 if x < 0
      mask Display: plot(-50,-50,50,50,[-50,50],[0,0],[0,0],[-50,50],[-40,0],[-30,-30],[0,40],[30,30])
  Out1 : Outport  InitialOutput=0
  wires:
  direction1/1(out_1) -> Out1/1
  In1/1 -> Abs2/1
  Abs2/1 -> direction1/1(in_1)

== system OMSv1_3/OMS v1.3  03/28/07/IM CN-LMLN/NI Control/DZ .5 ==
  note: We just output zero when the dead zone is in effect, and leave the
      |  output alone the rest of the time.
  note: This block is a better implementation of a dead zone than  the
      | block supplied by SIMULINK, because here we don't _subtract_
      | the dead zone from the rest of output.
  in_1 : Inport
  Abs : Abs  Orientation=down  SaturateOnIntegerOverflow=on
  Relational Operator : RelationalOperator  InputSameDT=on
  Switch6 : Switch  Threshold=.5  SaturateOnIntegerOverflow=on  InputSameDT=on
  dead zone : Constant  Orientation=up  Value=.5
  pos (deg) criterion1 : Constant  Orientation=left  Value=0
  out_1 : Outport  InitialOutput=0
  wires:
  Relational Operator/1 -> Switch6/2
  dead zone/1 -> Relational Operator/2
  pos (deg) criterion1/1 -> Switch6/3
  Abs/1 -> Relational Operator/1
  in_1/1 -> Switch6/1, Abs/1
  Switch6/1 -> out_1/1

== system OMSv1_3/OMS v1.3  03/28/07/IM CN-LMLN/NI Control/Latch1 ==
  in_1 : Inport
  in_2 : Inport  Port=2
  Demux : Demux  Outputs=2
  Logic : CombinatorialLogic  TruthTable=[0 1;0 1;1 0;0 1;1 0;0 1;1 0;1 0]
  Memory : Memory  Orientation=left  X0=ini
  Mux : Mux  Inputs=3
  out_1 : Outport  InitialOutput=0
  out_2 : Outport  Port=2  InitialOutput=0
  wires:
  in_2/1 -> Mux/3
  in_1/1 -> Mux/2
  Memory/1 -> Mux/1
  Demux/1 -> out_1/1, Memory/1
  Mux/1 -> Logic/1
  Logic/1 -> Demux/1
  Demux/2 -> out_2/1

== system OMSv1_3/OMS v1.3  03/28/07/IM CN-LMLN/NI Control/Latch2 ==
  in_1 : Inport
  in_2 : Inport  Port=2
  Demux : Demux  Outputs=2
  Logic : CombinatorialLogic  TruthTable=[0 1;0 1;1 0;0 1;1 0;0 1;1 0;1 0]
  Memory : Memory  Orientation=left  X0=ini
  Mux : Mux  Inputs=3
  out_1 : Outport  InitialOutput=0
  out_2 : Outport  Port=2  InitialOutput=0
  wires:
  Demux/2 -> out_2/1
  Logic/1 -> Demux/1
  Mux/1 -> Logic/1
  Demux/1 -> Memory/1, out_1/1
  Memory/1 -> Mux/1
  in_1/1 -> Mux/2
  in_2/1 -> Mux/3

== system OMSv1_3/OMS v1.3  03/28/07/IM CN-LMLN/NI Control/Zero-Cross ==
  note: Zero Cross Detect
  "[epr]" : Inport
  Relational Operator : RelationalOperator  Operator=~=  InputSameDT=on
  Sign2 : Subsystem
      mask Type: Sign
      mask Description: y = sign(x)
      mask Help: Sign Function:\n\t\t\ty = 1 if x > 0\n\t\t\ty = 0 if x = 0\n\t\t\ty = -1 if x < 0
      mask Display: plot(-50,-50,50,50,[-50,50],[0,0],[0,0],[-50,50],[-40,0],[-30,-30],[0,40],[30,30])
  loop breaker1 : Memory
  "[epneq]" : Outport  InitialOutput=0
  wires:
  Relational Operator/1 -> "[epneq]"/1
  loop breaker1/1 -> Relational Operator/2
  "[epr]"/1 -> Sign2/1(in_1)
  Sign2/1(out_1) -> Relational Operator/1, loop breaker1/1

== system OMSv1_3/OMS v1.3  03/28/07/IM CN-LMLN/NI Control/leading edge detect ==
  note: leading edge detection
  in_1 : Inport
  Abs : Abs  SaturateOnIntegerOverflow=on
  Derivative : Derivative
  Relational Operator : RelationalOperator  Operator===  InputSameDT=on
  Sign : Subsystem
      mask Type: Sign
      mask Description: y = sign(x)
      mask Help: Sign Function:\n\t\t\ty = 1 if x > 0\n\t\t\ty = 0 if x = 0\n\t\t\ty = -1 if x < 0
      mask Display: plot(-50,-50,50,50,[-50,50],[0,0],[0,0],[-50,50],[-40,0],[-30,-30],[0,40],[30,30])
  Threshold 1 : Constant
  out_1 : Outport  InitialOutput=0
  wires:
  in_1/1 -> Abs/1
  Relational Operator/1 -> out_1/1
  Threshold 1/1 -> Relational Operator/2
  Sign/1(out_1) -> Relational Operator/1
  Derivative/1 -> Sign/1(in_1)
  Abs/1 -> Derivative/1

== system OMSv1_3/OMS v1.3  03/28/07/IM CN-LMLN/NI Control/leading edge detect1 ==
  note: leading edge detection
  in_1 : Inport
  Abs : Abs  SaturateOnIntegerOverflow=on
  Derivative : Derivative
  Relational Operator : RelationalOperator  Operator===  InputSameDT=on
  Sign : Subsystem
      mask Type: Sign
      mask Description: y = sign(x)
      mask Help: Sign Function:\n\t\t\ty = 1 if x > 0\n\t\t\ty = 0 if x = 0\n\t\t\ty = -1 if x < 0
      mask Display: plot(-50,-50,50,50,[-50,50],[0,0],[0,0],[-50,50],[-40,0],[-30,-30],[0,40],[30,30])
  Threshold 1 : Constant
  out_1 : Outport  InitialOutput=0
  wires:
  Abs/1 -> Derivative/1
  Derivative/1 -> Sign/1(in_1)
  Sign/1(out_1) -> Relational Operator/1
  Threshold 1/1 -> Relational Operator/2
  Relational Operator/1 -> out_1/1
  in_1/1 -> Abs/1

== system OMSv1_3/OMS v1.3  03/28/07/IM CN-LMLN/NI Control/trailing edge detect ==
  note: It is also possible to remove the SIGNUM function
      | and the '==', and replace them with a simple
      | switch with a threshold of (say) 150 or so.
  note: trailing edge detection
  in_1 : Inport
  Abs : Abs  SaturateOnIntegerOverflow=on
  Derivative : Derivative
  Relational Operator : RelationalOperator  Operator===  InputSameDT=on
  Sign : Subsystem
      mask Type: Sign
      mask Description: y = sign(x)
      mask Help: Sign Function:\n\t\t\ty = 1 if x > 0\n\t\t\ty = 0 if x = 0\n\t\t\ty = -1 if x < 0
      mask Display: plot(-50,-50,50,50,[-50,50],[0,0],[0,0],[-50,50],[-40,0],[-30,-30],[0,40],[30,30])
  Threshold 1 : Constant  Value=-1
  out_1 : Outport  InitialOutput=0
  wires:
  Abs/1 -> Derivative/1
  Derivative/1 -> Sign/1(in_1)
  Sign/1(out_1) -> Relational Operator/1
  Threshold 1/1 -> Relational Operator/2
  Relational Operator/1 -> out_1/1
  in_1/1 -> Abs/1

== system OMSv1_3/OMS v1.3  03/28/07/IM CN-LMLN/Sacc Blank/Latch1 ==
  in_1 : Inport
  in_2 : Inport  Port=2
  Demux : Demux  Outputs=2
  Logic : CombinatorialLogic  TruthTable=[0 1;0 1;1 0;0 1;1 0;0 1;1 0;1 0]
  Memory : Memory  Orientation=left  X0=ini
  Mux : Mux  Inputs=3
  out_1 : Outport  InitialOutput=0
  out_2 : Outport  Port=2  InitialOutput=0
  wires:
  Demux/2 -> out_2/1
  Logic/1 -> Demux/1
  Mux/1 -> Logic/1
  Demux/1 -> out_1/1, Memory/1
  Memory/1 -> Mux/1
  in_1/1 -> Mux/2
  in_2/1 -> Mux/3

== system OMSv1_3/OMS v1.3  03/28/07/IM CN-LMLN/Sacc Blank/Latch2 ==
  in_1 : Inport
  in_2 : Inport  Port=2
  Demux : Demux  Outputs=2
  Logic : CombinatorialLogic  TruthTable=[0 1;0 1;1 0;0 1;1 0;0 1;1 0;1 0]
  Memory : Memory  Orientation=left  X0=ini
  Mux : Mux  Inputs=3
  out_1 : Outport  InitialOutput=0
  out_2 : Outport  Port=2  InitialOutput=0
  wires:
  in_2/1 -> Mux/3
  in_1/1 -> Mux/2
  Memory/1 -> Mux/1
  Demux/1 -> Memory/1, out_1/1
  Mux/1 -> Logic/1
  Logic/1 -> Demux/1
  Demux/2 -> out_2/1
